simulink model "impresora"  (R2020b)
settings: Solver=VariableStepAuto  StartTime=0.0  StopTime=20  RelTol=1e-3
libraries: fuzblock x1
settings Model: Creator=snopv  LastModifiedBy=snopv

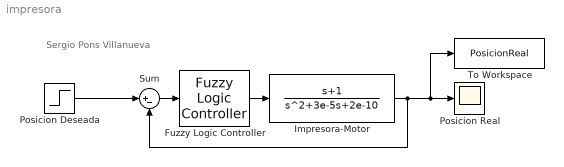
== system impresora ==
  note: Sergio Pons Villanueva
  Fuzzy Logic Controller : fuzblock/Fuzzy Logic  Controller  FIS=Impresora  OutputSampleNumber=101  DataType=double  FuzzifiedInputs=off  RuleFiringStrengths=off  RuleOutputs=off  AggregatedOutputs=off  SimulateUsing=Interpreted execution  OutOfRangeInputValueMessage=warning  NoRuleFiredMessage=warning  EmptyOutputFuzzySetMessage=warning
  Impresora-Motor : TransferFcn  Numerator=[1 1]  Denominator=[1 3e-5 2e-10]
  Posicion Deseada : Step  Time=0  After=0.1  SampleTime=0
  Posicion Real : Scope
  Sum : Sum  Inputs=|+-
  To Workspace : ToWorkspace  VariableName=PosicionReal  SaveFormat=Timeseries  SampleTime=-1
  wires:
  Fuzzy Logic Controller/1 -> Impresora-Motor/1
  Sum/1 -> Fuzzy Logic Controller/1
  Posicion Deseada/1 -> Sum/1
  Impresora-Motor/1 -> Sum/2, To Workspace/1, Posicion Real/1
